simulink model "tutor_pidma"  (Simulink 5.0)
settings: Solver=FixedStepDiscrete  StartTime=0.0  StopTime=500.0  FixedStep=0.1  RelTol=1e-3
libraries: mathlib x5, reglib x4, execlib x2, genlib x2, arclib x1
settings Model: LastModifiedBy=david  ExtModeTrigMode=oneshot  ExtModeArmWhenConnect=off  LimitDataPoints=off  BooleanDataType=off

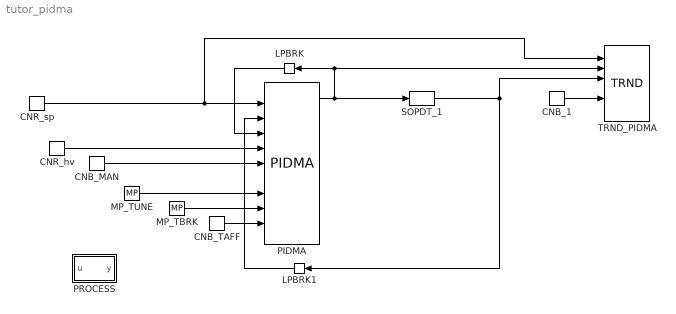
== system tutor_pidma ==
  CNB_1 : mathlib/CNB  YCN=on
  CNB_MAN : mathlib/CNB  YCN=on
  CNB_TAFF : mathlib/CNB  YCN=on
  CNR_hv : mathlib/CNR  ycn=0
  CNR_sp : mathlib/CNR  ycn=0.5
  LPBRK : execlib/LPBRK  Orientation=left
  LPBRK1 : execlib/LPBRK  Orientation=left
  MP_TBRK : genlib/MP  pwidth=1  BSTATE=off  RPTF=off
  MP_TUNE : genlib/MP  pwidth=1  BSTATE=off  RPTF=off
  PIDMA : reglib/PIDMA  irtype=6  RACT=off  k=1  ti=5.5  td=0  nd=4  b=1  c=0  tt=1  hilim=1  lolim=-1  dz=0  icotype=1  ittype=7  iainf=1  DGC=off  tdg=1  tn=2  amp=0.2  dy=0.1  ispeed=2  ipid=1
  PROCESS : Subsystem  mask(REX sequence){kp=}
      mask prompts: kp "process_gain"
  SOPDT_1 : reglib/SOPDT  itf=3  k0=10  tau=0  tau1=1  tau2=1  om=0.2  ksi=0.6  del=0  pb0=1  pb1=1  pa0=1  pa1=1
  TRND_PIDMA : arclib/TRND  n=3  l=100  btype=8  ptype1=1: Store  ptype2=1: Store  ptype3=1: Store  ptype4=1: Store  pfac=1  afac=0  arc=0  id=1  Title=Trend Title
  wires:
  CNB_1/1 -> TRND_PIDMA/5
  CNB_MAN/1 -> PIDMA/6
  CNB_TAFF/1 -> PIDMA/10
  CNR_hv/1 -> PIDMA/5
  CNR_sp/1 -> PIDMA/2, TRND_PIDMA/1
  LPBRK/1 -> PIDMA/4
  LPBRK1/1 -> PIDMA/3
  MP_TBRK/1 -> PIDMA/9
  MP_TUNE/1 -> PIDMA/8
  PIDMA/1 -> SOPDT_1/1, LPBRK/1, TRND_PIDMA/2
  SOPDT_1/1 -> LPBRK1/1, TRND_PIDMA/3

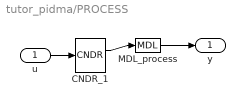
== system tutor_pidma/PROCESS ==
  CNDR_1 : reglib/CNDR  n=2  SATF=off  up=[-2.0 2.0]  yp=[-2.0 2.0]
  MDL_process : reglib/MDL  k0=kp  del=2  tau1=5  tau2=2
  u : Inport  Port=1
  y : Outport  Port=1
  wires:
  CNDR_1/1 -> MDL_process/1
  MDL_process/1 -> y/1
  u/1 -> CNDR_1/1
